simulink model "unicycle_simulink"  (R2020b)
settings: Solver=VariableStepAuto  StartTime=0.0  StopTime=50  RelTol=1e-3
values from neighbouring files (symbols this model uses):
  init_heading = b(end)    [checking_simulink_with_matlab.m]    (also in lloyd_wtd_adaptive_nonconvex.m = init_heading_list(i); lloyd_wtd_unicycle.m = init_heading_list(i))
libraries: simulink x3, robotmobilelib x1
settings Model: Creator=nijil  LastModifiedBy=nijil

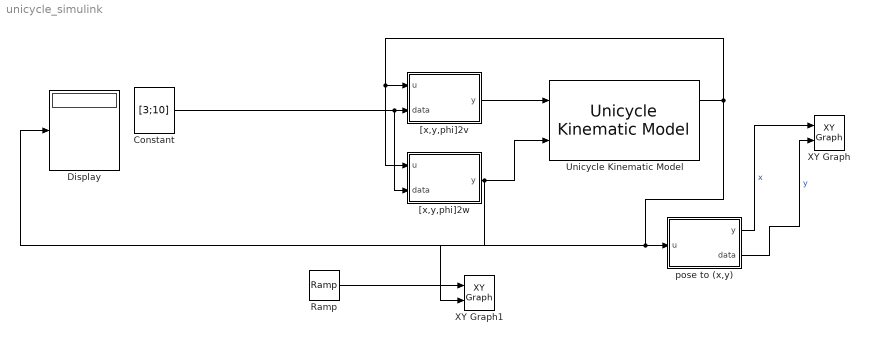
== system unicycle_simulink ==
  Constant : Constant  Value=[3;10]  VectorParams1D=off
  Display : Display
  Ramp : simulink/Sources/Ramp  slope=1  start=0  InitialOutput=0
  Unicycle Kinematic Model : robotmobilelib/Unicycle Kinematic Model  VehicleInputs=Vehicle Speed & Heading Angular Velocity  WheelRadius=0.1  WheelSpeedRange=[-pi pi]  InitialState=[0 0 init_heading]  SimulateUsing=Interpreted execution
      settings: SourceProductBaseCode=RO
  XY Graph : simulink/Sinks/XY Graph  xmin=-10  xmax=10  ymin=-10  ymax=10  st=-1
  XY Graph1 : simulink/Sinks/XY Graph  xmin=0  xmax=50  ymin=-10  ymax=10  st=-1
  "[x,y,phi]2v" : MATLAB Function  TreatAsAtomicUnit=on
  "[x,y,phi]2w" : MATLAB Function  TreatAsAtomicUnit=on
  pose to (x,y) : MATLAB Function  TreatAsAtomicUnit=on
  wires:
  "[x,y,phi]2v"/1(y) -> Unicycle Kinematic Model/1
  "[x,y,phi]2w"/1(y) -> XY Graph1/2, Unicycle Kinematic Model/2
  pose to (x,y)/1(y) -> XY Graph/1  "x"
  pose to (x,y)/2(data) -> XY Graph/2  "y"
  Ramp/1 -> XY Graph1/1
  Constant/1 -> "[x,y,phi]2w"/2(data), "[x,y,phi]2v"/2(data)
  Unicycle Kinematic Model/1 -> "[x,y,phi]2w"/1(u), "[x,y,phi]2v"/1(u), pose to (x,y)/1(u), Display/1

== matlab function unicycle_simulink/[x,y,phi]2v ==
  data: u input; y output; data input
function y = fcn(u, data)
fd=[data(1)-u(1) data(2)-u(2)];
hi=[cos(u(3)) sin(u(3))];
% hip=[-sin(u(3)) cos(u(3))];
y = norm(hi.*(hi*fd'),2);

== matlab function unicycle_simulink/pose to (x,y) ==
  data: u input; y output; data output
function [y,data] = fcn(u)
y=u(1);
data = u(2);

== matlab function unicycle_simulink/[x,y,phi]2w ==
  data: u input; y output; data input
function y = fcn(u, data)
fd=[data(1)-u(1) data(2)-u(2)];
% hi=[cos(u(3)) sin(u(3))];
hip=[-sin(u(3)) cos(u(3))];
y =(hip*fd');
